simulink model "Series_Resonance_Converter_with_transformer"  (R2022b)
settings: Solver=ode23t  StartTime=0.0  StopTime=.1  MaxStep=1e-7  RelTol=1e-3
undefined symbols (not defined in the file): DiscIntNeverNeededParam
libraries: spsSeriesRLCBranchLib x6, spsDiodeLib x4, spsMosfetLib x4, spsOnDelayLib x4, spsCurrentMeasurementLib x3, slpidlib x2, spsDCVoltageSourceLib x1, spsLinearTransformerLib x1, simulink x1, spsVoltageMeasurementLib x1, sps_lib x1
settings Model: Creator=es-ahmedabdellatif20  LastModifiedBy=es-ahmedabdellatif20

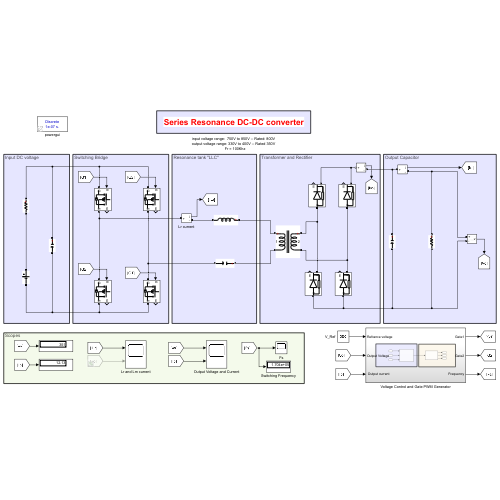
[thumbnail: Simulink's stored preview of the top-level diagram]
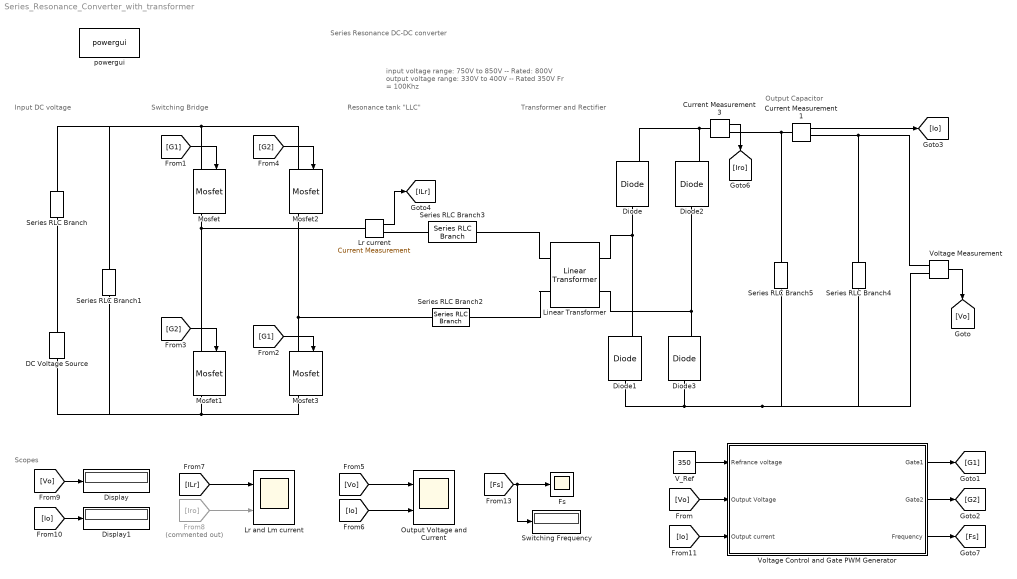
== system Series_Resonance_Converter_with_transformer ==
  note: input voltage range: 750V to 850V -- Rated: 800V
      | output voltage range: 330V to 400V -- Rated 350V
      | Fr = 100Khz
  note: Scopes
  note: Input DC voltage
  note: Output Capacitor
  note: Transformer and Rectifier
  note: Resonance tank "LLC"
  note: Switching Bridge
  note: Series Resonance DC-DC converter
  Current Measurement1 : spsCurrentMeasurementLib/Current Measurement  PhasorSimulation=off  OutputType=Complex  PSBequivalent=0
  Current Measurement3 : spsCurrentMeasurementLib/Current Measurement  PhasorSimulation=off  OutputType=Complex  PSBequivalent=0
  DC Voltage Source : spsDCVoltageSourceLib/DC Voltage Source  Amplitude=820  Measurements=None
  Diode{,1..3} (4 alike) : spsDiodeLib/Diode  Ron=0.001  Lon=0  Vf=0.8  IC=0  UseSnubber=0  Rs=500  Cs=250e-9  Measurements=on
  Display : Display
  Display1 : Display
  From8 : From  Commented=on  GotoTag=Iro
  Fs : Scope
  Linear Transformer : spsLinearTransformerLib/Linear Transformer  UNITS=SI  NominalPower=[ 10000 200000 ]  winding1=[800 404e-3 0]  winding2=[400 404e-3 0]  ThreeWindings=off  winding3=[3.15e+05 0.7938 0.084225]  RmLm=[1.0804e+06 4.85e-3]  Measurements=None  DataType=on
  Lr and Lm current : Scope  NumInputPorts=2
  Lr current : spsCurrentMeasurementLib/Current Measurement  PhasorSimulation=off  OutputType=Complex  PSBequivalent=0
  Mosfet{,1..3} (4 alike) : spsMosfetLib/Mosfet  Ron=0.1  Lon=0  Rd=0.01  Vfd=0  IC=0  Rs=1e5  Cs=inf  Measurements=on
  Output Voltage and Current : Scope  NumInputPorts=2
  Series RLC Branch : spsSeriesRLCBranchLib/Series RLC Branch  LConnTagsString=__new0  RConnTagsString=__new0  BranchType=R  Resistance=.001  Inductance=1e-3  SetiL0=off  InitialCurrent=0  Capacitance=1e-6  Setx0=off  InitialVoltage=0  Measurements=None
  Series RLC Branch1 : spsSeriesRLCBranchLib/Series RLC Branch  LConnTagsString=__new0  RConnTagsString=__new0  BranchType=C  Resistance=.001  Inductance=1e-3  SetiL0=off  InitialCurrent=0  Capacitance=660e-6  Setx0=off  InitialVoltage=0  Measurements=None
  Series RLC Branch2 : spsSeriesRLCBranchLib/Series RLC Branch  LConnTagsString=__new0  RConnTagsString=__new0  BranchType=C  Resistance=.001  Inductance=1e-3  SetiL0=off  InitialCurrent=0  Capacitance=66e-09  Setx0=off  InitialVoltage=0  Measurements=None
  Series RLC Branch3 : spsSeriesRLCBranchLib/Series RLC Branch  LConnTagsString=__new0  RConnTagsString=__new0  BranchType=L  Resistance=.001  Inductance=3.6e-05  SetiL0=off  InitialCurrent=10e-3  Capacitance=660e-6  Setx0=off  InitialVoltage=0  Measurements=None
  Series RLC Branch4 : spsSeriesRLCBranchLib/Series RLC Branch  LConnTagsString=__new0  RConnTagsString=__new0  BranchType=R  Resistance=28.928  Inductance=1e-3  SetiL0=off  InitialCurrent=0  Capacitance=600e-6  Setx0=on  InitialVoltage=400  Measurements=None
  Series RLC Branch5 : spsSeriesRLCBranchLib/Series RLC Branch  LConnTagsString=__new0  RConnTagsString=__new0  BranchType=C  Resistance=.001  Inductance=1e-3  SetiL0=off  InitialCurrent=0  Capacitance=600e-6  Setx0=on  InitialVoltage=0  Measurements=None
  Switching Frequency : Display
  V_Ref : Constant  Value=350
  Voltage Control and Gate PWM Generator : Subsystem
  Voltage Measurement : spsVoltageMeasurementLib/Voltage Measurement  PhasorSimulation=off  OutputType=Complex  PSBequivalent=0
  powergui : sps_lib/powergui  Priority=1  SimulationMode=Discrete  SampleTime=1e-7  frequency=60  Iterations=50  frequencyindice=0  Pbase=100e6  ErrMax=1e-4  UnitsV=kV  UnitsW=MW  buscounter=0  FunctionMessages=off  echomessages=off  EnableUseOfTLC=off  CurrentSourceSwitches=off  DisableSnubberDevices=off  DisableRonSwitches=off  DisableVfSwitches=off  DisplayEquations=off  AutomaticDiscreteSolvers=off  SolverType=Tustin/Backward Euler (TBE)  Interpol=off  ExternalGateDelay=off  methode=off  Ts=100  x0status=blocks  SPID=on  SwTol=0  HookPort=off  NonlinearTolerance=1e-4  nMaxIteration=100  ContinueOnMaxIteration=off  RestoreLinks=warning  ResistiveCurrentMeasurement=off  Frange=[0:2:500]  Ylog=off  Xlog=on  ShowGrid=off  save=off  variable=ZData  structure=0  ZoomFFT=off  StartTime=0.0  cycles=1  DisplayStyle=1  fundamental=60  FreqAxis=off  MaxFrequency=1000  frequencyindicesteady=1  RmsSteady=1  display=off
  wires:
  Voltage Measurement/1 -> [Vo]
  [Vo] -> Voltage Control and Gate PWM Generator/2(Output Voltage)
  V_Ref/1 -> Voltage Control and Gate PWM Generator/1(Refrance voltage)
  Voltage Control and Gate PWM Generator/1(Gate1) -> [G1]
  Voltage Control and Gate PWM Generator/2(Gate2) -> [G2]
  [G1] -> Mosfet/1
  [G1] -> Mosfet3/1
  [G2] -> Mosfet1/1
  [G2] -> Mosfet2/1
  Current Measurement1/1 -> [Io]
  Lr current/1 -> [ILr]
  [Vo] -> Output Voltage and Current/1
  [Io] -> Output Voltage and Current/2
  From8/1 -> Lr and Lm current/2
  [ILr] -> Lr and Lm current/1
  [Io] -> Display1/1
  [Vo] -> Display/1
  Current Measurement3/1 -> [Iro]
  [Io] -> Voltage Control and Gate PWM Generator/3(" Output current")
  Voltage Control and Gate PWM Generator/3(Frequency) -> [Fs]
  [Fs] -> Fs/1, Switching Frequency/1
  connections:
  Linear Transformer/LConn2 -- Series RLC Branch2/LConn1
  Mosfet2/LConn1 -- Series RLC Branch/LConn1 -- Series RLC Branch1/LConn1 -- Mosfet/LConn1
  Mosfet/RConn1 -- Mosfet1/LConn1 -- Lr current/LConn1
  Mosfet1/RConn1 -- DC Voltage Source/LConn1 -- Series RLC Branch1/RConn1 -- Mosfet3/RConn1
  DC Voltage Source/RConn1 -- Series RLC Branch/RConn1
  Diode1/RConn1 -- Linear Transformer/RConn1 -- Diode/LConn1
  Diode2/LConn1 -- Linear Transformer/RConn2 -- Diode3/RConn1
  Diode3/LConn1 -- Series RLC Branch5/RConn1 -- Series RLC Branch4/RConn1 -- Voltage Measurement/LConn2 -- Diode1/LConn1
  Diode2/RConn1 -- Diode/RConn1 -- Current Measurement3/LConn1
  Series RLC Branch3/LConn1 -- Linear Transformer/LConn1
  Voltage Measurement/LConn1 -- Current Measurement1/RConn1 -- Series RLC Branch4/LConn1
  Series RLC Branch5/LConn1 -- Current Measurement3/RConn1 -- Current Measurement1/LConn1
  Series RLC Branch2/RConn1 -- Mosfet2/RConn1 -- Mosfet3/LConn1
  Lr current/RConn1 -- Series RLC Branch3/RConn1

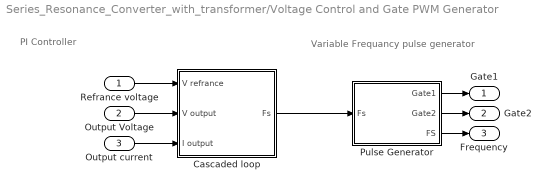
== system Series_Resonance_Converter_with_transformer/Voltage Control and Gate PWM Generator ==
  note: PI Controller
  note: Variable Frequancy pulse generator
  Refrance voltage : Inport
  Output Voltage : Inport  Port=2
  " Output current" : Inport  Port=3
  Cascaded loop : Subsystem
  Pulse Generator : Subsystem
  Gate1 : Outport
  Gate2 : Outport  Port=2
  Frequency : Outport  Port=3
  wires:
  Pulse Generator/3(FS) -> Frequency/1
  Pulse Generator/1(Gate1) -> Gate1/1
  Pulse Generator/2(Gate2) -> Gate2/1
  Refrance voltage/1 -> Cascaded loop/1(V refrance)
  Output Voltage/1 -> Cascaded loop/2(V output)
  " Output current"/1 -> Cascaded loop/3(I output)
  Cascaded loop/1(Fs) -> Pulse Generator/1(Fs)

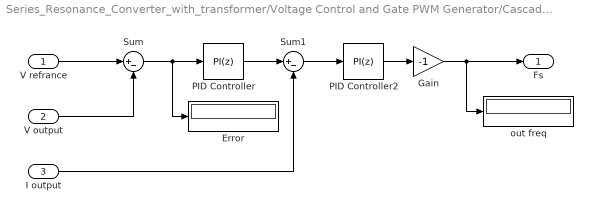
== system Series_Resonance_Converter_with_transformer/Voltage Control and Gate PWM Generator/Cascaded loop ==
  V refrance : Inport
  V output : Inport  Port=2
  I output : Inport  Port=3
  Error : Display
  Gain : Gain  Gain=-1
  PID Controller : slpidlib/PID Controller  Controller=PI  Form=Parallel  TimeDomain=Discrete-time  UseExternalTs=off  SampleTime=1e-7  IntegratorMethod=Forward Euler  FilterMethod=Forward Euler  ControllerParametersSource=internal  P=6  I=20.1  UseKiTs=off  D=0  N=100  UseFilter=on  TunerSelectOption=Transfer Function Based (PID Tuner App)  InitialConditionSource=internal  InitialConditionForIntegrator=0  InitialConditionForFilter=0  DifferentiatorICPrevScaledInput=0  ExternalReset=none  TrackingMode=off  Kt=1  LimitOutput=off  SatLimitsSource=internal  UpperSaturationLimit=inf  LowerSaturationLimit=-inf  LinearizeAsGain=on  AntiWindupMode=none  Kb=1  LimitIntegrator=off  UpperIntegratorSaturationLimit=inf  LowerIntegratorSaturationLimit=-inf  POutMin=[]  POutMax=[]  IOutMin=[]  IOutMax=[]  DOutMin=[]  DOutMax=[]  NOutMin=[]  NOutMax=[]  SumOutMin=[]  SumOutMax=[]  SaturationOutMin=[]  SaturationOutMax=[]  PParamMin=[]  PParamMax=[]  IParamMin=[]  IParamMax=[]  DParamMin=[]  DParamMax=[]  NParamMin=[]  NParamMax=[]  KbParamMin=[]  KbParamMax=[]  KtParamMin=[]  KtParamMax=[]  KbOutMin=[]  KbOutMax=[]  KtOutMin=[]  KtOutMax=[]  IntegratorOutMin=[]  IntegratorOutMax=[]  FilterOutMin=[]  FilterOutMax=[]  SumI1OutMin=[]  SumI1OutMax=[]  SumI2OutMin=[]  SumI2OutMax=[]  SumI3OutMin=[]  SumI3OutMax=[]  SumI4OutMin=[]  SumI4OutMax=[]  SumDOutMin=[]  SumDOutMax=[]  DifferentiatorOutMin=[]  DifferentiatorOutMax=[]  FilterDiffOutCoefMin=[]  FilterDiffOutCoefMax=[]  ReciprocalOutMin=[]  ReciprocalOutMax=[]  SumDenOutMin=[]  SumDenOutMax=[]  SumNumOutMin=[]  SumNumOutMax=[]  DivideOutMin=[]  DivideOutMax=[]  UdiffTsProdOutMin=[]  UdiffTsProdOutMax=[]  NTsProdOutMin=[]  NTsProdOutMax=[]  UintegralTsProdOutMin=[]  UintegralTsProdOutMax=[]  UngainTsProdOutMin=[]  UngainTsProdOutMax=[]  ClampingZeroOutDataTypeStr=Inherit: Inherit via back propagation  ClampingZeroOutMin=[]  ClampingZeroOutMax=[]  FilterDenConstantOutDataTypeStr=Inherit: Inherit via back propagation  FilterDenConstantOutMin=[]  FilterDenConstantOutMax=[]  PCopyOutDataTypeStr=Inherit: Inherit via back propagation  PCopyOutMin=[]  PCopyOutMax=[]  NCopyOutDataTypeStr=Inherit: Inherit via back propagation  NCopyOutMin=[]  NCopyOutMax=[]  IntegratorContinuousStateAttributes=''  IntegratorStateMustResolveToSignalObject=off  IntegratorRTWStateStorageClass=Auto  FilterContinuousStateAttributes=''  FilterStateMustResolveToSignalObject=off  FilterRTWStateStorageClass=Auto  ParallelPVariant=InternalParameters  IdealPVariant=Disabled  IVariant=InternalParameters  DVariant=Disabled  IntegratorVariant=Discrete  SatVariant=Disabled  AWVariant=Passthrough  PCopyVariant=Disabled  TRVariant=Disabled  FdbkBlocksVariant=Forward  IdealPFdbkVariant=Disabled  SatFdbkVariant=Disabled  DerivativeFilterVariant=Disabled  NVariant=Disabled  NCopyVariant=Disabled_SignalSpec  FilterICVariant=Disabled  IntegratorICVariant=InternalICs  ExternalResetVariant=Disabled  TRSumVariant=Passthrough  SumFdbkVariant=Disabled  SumVariant=Sum_PI  TsampFilterVariant=InternalTs  TsampNgainVariant=Passthrough  TsampIntegralVariant=Passthrough  ExternalSaturationOutDataTypeStr=Inherit: Same as second input
  PID Controller2 : slpidlib/PID Controller  Controller=PI  Form=Parallel  TimeDomain=Discrete-time  UseExternalTs=off  SampleTime=1e-7  IntegratorMethod=Forward Euler  FilterMethod=Forward Euler  ControllerParametersSource=internal  P=10  I=10000  UseKiTs=off  D=0  N=100  UseFilter=on  TunerSelectOption=Transfer Function Based (PID Tuner App)  InitialConditionSource=internal  InitialConditionForIntegrator=-200e3  InitialConditionForFilter=0  DifferentiatorICPrevScaledInput=0  ExternalReset=none  IgnoreLimit=on  TrackingMode=off  Kt=1  LimitOutput=on  SatLimitsSource=internal  UpperSaturationLimit=-70e3  LowerSaturationLimit=-200e3  LinearizeAsGain=on  AntiWindupMode=none  Kb=1  LimitIntegrator=off  UpperIntegratorSaturationLimit=inf  LowerIntegratorSaturationLimit=-inf  POutMin=[]  POutMax=[]  IOutMin=[]  IOutMax=[]  DOutMin=[]  DOutMax=[]  NOutMin=[]  NOutMax=[]  SumOutMin=[]  SumOutMax=[]  SaturationOutMin=[]  SaturationOutMax=[]  PParamMin=[]  PParamMax=[]  IParamMin=[]  IParamMax=[]  DParamMin=[]  DParamMax=[]  NParamMin=[]  NParamMax=[]  KbParamMin=[]  KbParamMax=[]  KtParamMin=[]  KtParamMax=[]  KbOutMin=[]  KbOutMax=[]  KtOutMin=[]  KtOutMax=[]  IntegratorOutMin=[]  IntegratorOutMax=[]  FilterOutMin=[]  FilterOutMax=[]  SumI1OutMin=[]  SumI1OutMax=[]  SumI2OutMin=[]  SumI2OutMax=[]  SumI3OutMin=[]  SumI3OutMax=[]  SumI4OutMin=[]  SumI4OutMax=[]  SumDOutMin=[]  SumDOutMax=[]  DifferentiatorOutMin=[]  DifferentiatorOutMax=[]  FilterDiffOutCoefMin=[]  FilterDiffOutCoefMax=[]  ReciprocalOutMin=[]  ReciprocalOutMax=[]  SumDenOutMin=[]  SumDenOutMax=[]  SumNumOutMin=[]  SumNumOutMax=[]  DivideOutMin=[]  DivideOutMax=[]  UdiffTsProdOutMin=[]  UdiffTsProdOutMax=[]  NTsProdOutMin=[]  NTsProdOutMax=[]  UintegralTsProdOutMin=[]  UintegralTsProdOutMax=[]  UngainTsProdOutMin=[]  UngainTsProdOutMax=[]  ClampingZeroOutDataTypeStr=Inherit: Inherit via back propagation  ClampingZeroOutMin=[]  ClampingZeroOutMax=[]  FilterDenConstantOutDataTypeStr=Inherit: Inherit via back propagation  FilterDenConstantOutMin=[]  FilterDenConstantOutMax=[]  PCopyOutDataTypeStr=Inherit: Inherit via back propagation  PCopyOutMin=[]  PCopyOutMax=[]  NCopyOutDataTypeStr=Inherit: Inherit via back propagation  NCopyOutMin=[]  NCopyOutMax=[]  IntegratorContinuousStateAttributes=''  IntegratorStateMustResolveToSignalObject=off  IntegratorRTWStateStorageClass=Auto  FilterContinuousStateAttributes=''  FilterStateMustResolveToSignalObject=off  FilterRTWStateStorageClass=Auto  ParallelPVariant=InternalParameters  IdealPVariant=Disabled  IVariant=InternalParameters  DVariant=Disabled  IntegratorVariant=Discrete  SatVariant=Enabled  AWVariant=Passthrough  PCopyVariant=Disabled  TRVariant=Disabled  FdbkBlocksVariant=Forward  IdealPFdbkVariant=Disabled  SatFdbkVariant=Disabled  DerivativeFilterVariant=Disabled  NVariant=Disabled  NCopyVariant=Disabled_SignalSpec  FilterICVariant=Disabled  IntegratorICVariant=InternalICs  ExternalResetVariant=Disabled  TRSumVariant=Passthrough  SumFdbkVariant=Disabled  SumVariant=Sum_PI  TsampFilterVariant=InternalTs  TsampNgainVariant=Passthrough  TsampIntegralVariant=Passthrough  ExternalSaturationOutDataTypeStr=Inherit: Same as second input
  Sum : Sum  Inputs=|+-
  Sum1 : Sum  Inputs=|+-
  out freq : Display
  Fs : Outport
  wires:
  Sum/1 -> Error/1, PID Controller/1
  PID Controller/1 -> Sum1/1
  PID Controller2/1 -> Gain/1
  V refrance/1 -> Sum/1
  V output/1 -> Sum/2
  I output/1 -> Sum1/2
  Sum1/1 -> PID Controller2/1
  Gain/1 -> Fs/1, out freq/1

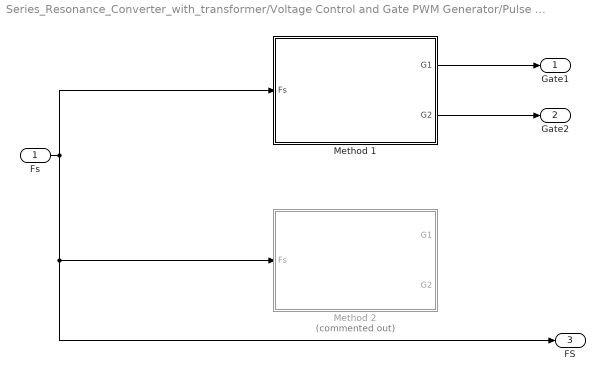
== system Series_Resonance_Converter_with_transformer/Voltage Control and Gate PWM Generator/Pulse Generator ==
  Fs : Inport
  Method 1 : Subsystem
  Method 2 : Subsystem  Commented=on
  Gate1 : Outport  VectorParamsAs1DForOutWhenUnconnected=off
  Gate2 : Outport  Port=2  VectorParamsAs1DForOutWhenUnconnected=off
  FS : Outport  Port=3  VectorParamsAs1DForOutWhenUnconnected=off
  wires:
  Method 1/1(G1) -> Gate1/1
  Method 1/2(G2) -> Gate2/1
  Fs/1 -> FS/1, Method 2/1(Fs), Method 1/1(Fs)

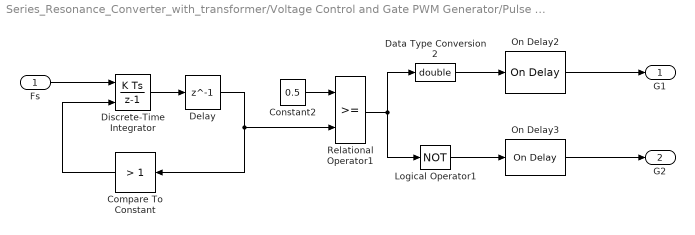
== system Series_Resonance_Converter_with_transformer/Voltage Control and Gate PWM Generator/Pulse Generator/Method 1 ==
  Fs : Inport
  Compare To Constant : simulink/Logic and Bit Operations/Compare To Constant  relop=>  const=1  OutDataTypeStr=boolean
  Constant2 : Constant  Value=0.5
  Data Type Conversion2 : DataTypeConversion  OutDataTypeStr=double  SaturateOnIntegerOverflow=off  RndMeth=Floor
  Delay : Delay  DelayLength=1  InitialCondition=0
  Discrete-Time Integrator : DiscreteIntegrator  ExternalReset=rising  SampleTime=-1  ICPrevOutput=DiscIntNeverNeededParam  ICPrevScaledInput=DiscIntNeverNeededParam
  Logical Operator1 : Logic  Operator=NOT  IconShape=distinctive  AllPortsSameDT=off  OutDataTypeStr=float('double')
  On Delay2 : spsOnDelayLib/On Delay  DelayType=On delay  delay=400e-9  ic=0  Ts=0
  On Delay3 : spsOnDelayLib/On Delay  DelayType=On delay  delay=400e-9  ic=0  Ts=0
  Relational Operator1 : RelationalOperator  OutDataTypeStr=boolean  InputSameDT=off
  G1 : Outport
  G2 : Outport  Port=2
  wires:
  Compare To Constant/1 -> Discrete-Time Integrator/2
  Relational Operator1/1 -> Data Type Conversion2/1, Logical Operator1/1
  Fs/1 -> Discrete-Time Integrator/1
  Delay/1 -> Relational Operator1/2, Compare To Constant/1
  Logical Operator1/1 -> On Delay3/1
  On Delay3/1 -> G2/1
  Discrete-Time Integrator/1 -> Delay/1
  Data Type Conversion2/1 -> On Delay2/1
  Constant2/1 -> Relational Operator1/1
  On Delay2/1 -> G1/1

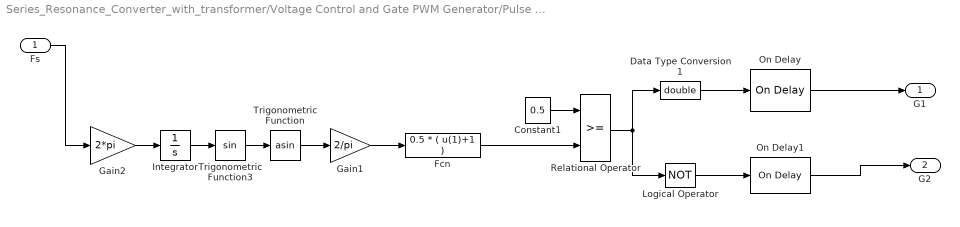
== system Series_Resonance_Converter_with_transformer/Voltage Control and Gate PWM Generator/Pulse Generator/Method 2 ==
  Fs : Inport
  Constant1 : Constant  Value=0.5
  Data Type Conversion1 : DataTypeConversion  OutDataTypeStr=double  SaturateOnIntegerOverflow=off  RndMeth=Floor
  Fcn : Fcn  Expr=0.5 * ( u(1)+1 )
  Gain1 : Gain  Gain=2/pi  SaturateOnIntegerOverflow=on  OutDataTypeStr=Inherit: Same as input  ParamDataTypeStr=Inherit: Same as input
  Gain2 : Gain  Gain=2*pi  SaturateOnIntegerOverflow=on  OutDataTypeStr=Inherit: Same as input  ParamDataTypeStr=Inherit: Same as input
  Integrator : Integrator
  Logical Operator : Logic  Operator=NOT  AllPortsSameDT=off  OutDataTypeStr=float('double')
  On Delay : spsOnDelayLib/On Delay  DelayType=On delay  delay=400e-9  ic=0  Ts=0
  On Delay1 : spsOnDelayLib/On Delay  DelayType=On delay  delay=400e-9  ic=0  Ts=0
  Relational Operator : RelationalOperator  OutDataTypeStr=boolean  InputSameDT=off
  Trigonometric Function : Trigonometry  Operator=asin
  Trigonometric Function3 : Trigonometry
  G1 : Outport
  G2 : Outport  Port=2
  wires:
  Logical Operator/1 -> On Delay1/1
  Integrator/1 -> Trigonometric Function3/1
  Gain2/1 -> Integrator/1
  Trigonometric Function3/1 -> Trigonometric Function/1
  Relational Operator/1 -> Logical Operator/1, Data Type Conversion1/1
  Constant1/1 -> Relational Operator/1
  Fcn/1 -> Relational Operator/2
  Trigonometric Function/1 -> Gain1/1
  Data Type Conversion1/1 -> On Delay/1
  Gain1/1 -> Fcn/1
  On Delay/1 -> G1/1
  Fs/1 -> Gain2/1
  On Delay1/1 -> G2/1
